simulink model "Model_14Bus_AC_DC_Microgrid"  (R2025a)
settings: Solver=ode23tb  StartTime=0.0  StopTime=0.1  MaxStep=1e-2  RelTol=1e-3
InitFcn:
  | Set_parameters_R2018
StopFcn:
  | Save_Data;
  | Graphics;
undefined symbols (not defined in the file): Clink, D1, Delta, dis1, dis10, dis11, dis12, dis13, dis14, dis2, dis3, dis4, dis5, dis6, dis7, dis8, dis9, Fc, Fnom, Hydride, Increment_MPPT, Ion, Ki_Ireg, Ki_VDCreg, Kp_Ireg, Kp_VDCreg, LimitL_Ireg, LimitL_VDCreg, Limits_MPPT, LimitU_Ireg, LimitU_VDCreg, Lithium, max_min, Metal, Nickel, P_Load_2, P_Load_3, Pnom, Pnom_T1, Pnom_T2, Pnom_T3, Pnom_xfo, Ql_Load_2, Ql_Load_3, R_Load_9, R_Load_DC, RL, Rl, RLff, Rls, sigbuilder_block, Ts, Ts_Control, Ts_Power, V1_LL_T3, Vf, Vfd, Vnom_dc, Vnom_DC, Vnom_Diesel ... (+5)
libraries: spsRMSLib x87, spsCurrentMeasurementLib x47, spsThreePhaseVIMeasurementLib x23, spsVoltageMeasurementLib x21, spsPowerLib x21, spsTHDLib x20, spsThreePhaseSeriesRLCBranchLib x20, spsSeriesRLCBranchLib x19, spsIGBTDiodeLib x14, spsThreePhaseBreakerLib x14, powerlib_extras x14, simulink x12
(part 3 of 9)

== system Model_14Bus_AC_DC_Microgrid/Bus_14 9 ==
  " r1_ L13" : Constant  Value=Rl
  Active powers losses A : Display
      settings: Format=bank
  Active powers losses B : Display
      settings: Format=bank
  Active powers losses c : Display
      settings: Format=bank
  "Delta Pabc " : Scope  NumInputPorts=4
      settings: SampleTime=Ts  Title=Active powers losses A (kW)  ActiveDisplayYMinimum=-0.00443  ActiveDisplayYMaximum=0.03985  DataLoggingSaveFormat=Array
  Math Function : Math  Operator=square  SignedPower=on
  Math Function1 : Math  Operator=square  SignedPower=on
  Math Function2 : Math  Operator=square  SignedPower=on
  Mux : Mux  Inputs=3
  Product : Product
  Product1 : Product
  Product2 : Product
  RMS1 : spsRMSLib/RMS  TrueRMS=on  Freq=60  RMSInit=0  Ts=0
  RMS2 : spsRMSLib/RMS  TrueRMS=on  Freq=60  RMSInit=0  Ts=0
  RMS3 : spsRMSLib/RMS  TrueRMS=on  Freq=60  RMSInit=0  Ts=0
  W_to_kW : Gain  Gain=1e-3
  W_to_kW1 : Gain  Gain=1e-3
  W_to_kW2 : Gain  Gain=1e-3
  tag scope: Power_Losse_abc_L8=global
  wires:
  Math Function/1 -> Product/2
  [Ia_L8] -> RMS2/1
  Math Function1/1 -> Product1/2
  [Ib_L8] -> RMS1/1
  Math Function2/1 -> Product2/2
  " r1_ L13"/1 -> Product2/1, Product1/1, Product/1
  [Ic_L8] -> RMS3/1
  Product/1 -> W_to_kW/1
  Product2/1 -> W_to_kW2/1
  Product1/1 -> W_to_kW1/1
  RMS2/1 -> Math Function/1
  RMS1/1 -> Math Function1/1
  RMS3/1 -> Math Function2/1
  W_to_kW/1 -> Mux/1, "Delta Pabc "/1, Active powers losses A/1  "D_Pa_kW"
  W_to_kW1/1 -> Mux/2, "Delta Pabc "/2, Active powers losses B/1  "D_Pb_kW"
  W_to_kW2/1 -> Active powers losses c/1, Mux/3, "Delta Pabc "/3  "D_Pc_kW"
  Mux/1 -> [Power_Losse_abc_L8], "Delta Pabc "/4

== system Model_14Bus_AC_DC_Microgrid/Bus_2 ==
  note: C
  note: B
  note: A
  note: A
  note: B
  note: Linea - Neutro
  note: C
  note: A
  note: B
  note: C
  Conv pu1 : Gain  Gain=sqrt (3) /Vnom_sec  SaturateOnIntegerOverflow=on  OutDataTypeStr=Inherit: Same as input  ParamDataTypeStr=Inherit: Same as input
  Conv pu2 : Gain  Gain=sqrt (3) /Vnom_sec  SaturateOnIntegerOverflow=on  OutDataTypeStr=Inherit: Same as input  ParamDataTypeStr=Inherit: Same as input
  Measurement1 : Scope  NumInputPorts=4
      settings: SampleTime=Ts  Title=Active Powers (W)  ActiveDisplayYMinimum=-7513.46294  ActiveDisplayYMaximum=8729.48723  DataLoggingVariableName=ScopeData7  DataLoggingSaveFormat=Array
  PLL : Subsystem
  PLL (3ph) : spsPLL3phLib/PLL (3ph)  Fmin=45  Par_Init=[0, 60]  ParK=[180, 3200, 1]  TcD=1e-4  MaxRateChangeFreq=12  FilterCutOffFreq=25  Ts=0  AGC=on
  Power Factor Block1 : Subsystem  mask(Power Factor Block){Freq=Fnom, Vinit=[0, 0], Iinit=[0, 0], Ts=0}
      mask prompts: Freq "Fundamental frequency (Hz):"; Vinit "Voltage initial input [ Mag, Phase (degrees) ]:"; Iinit "Current initial input [ Mag, Phase (degrees) ]:"; Ts "Sample time:"
      mask help:
      | Power Factor Block developed by Dr Rodney Tan
      | Version 1.01 (Aug 2016)
      |
      | Compute power factor and phase angle of AC circuit voltage-current pair at fundamental frequency.
      |
      | The computation is based on Power block and Complex number function block.
      |
      | For the first cycle of simulation, the outputs are held constant to the powers computed for the Voltage initial input and Current initial input parameters.
      mask Help:
      | <b>Fundamental Frequency (Hz)</b>
      | Specify the measurement fundamental frequency, in hertz, of the input signal.
      | 
      | <b>Voltage initial input [ Mag, Phase (degrees) ]</b>
      | Specify the voltage initial magnitude and phase to set a constant output for the first cycle of simulation.
      | 
      | <b>Current initial input [ Mag, Phase (degrees) ]</b>
      | Specify the current initial magnitude and phase to set a constant output for the first cycle of simulation.
      | 
      | <b>Sample Time</b>
      | Specify the sample time of the block, in seconds. Set to 0 to implement a continuous block.
      mask TypeOptions Freq: Power/Freq
      mask TypeOptions Vinit: Power/Vinit
      mask TypeOptions Iinit: Power/Iinit
      mask TypeOptions Ts: Power/Ts
  Power Factor1 : Display
  Scope : Scope
      settings: ActiveDisplayYMinimum=-60.00715  ActiveDisplayYMaximum=239.87716
  Scope2 : Scope
      settings: DataLoggingVariableName=ScopeData8
  THD : spsTHDLib/THD  Freq=60  Ts=Ts_Power
  THD (% and signal) : Scope  NumInputPorts=2
      settings: TimeSpan=0.1  ActiveDisplayYMinimum=-187.16352  ActiveDisplayYMaximum=186.2085  DataLoggingVariableName=ScopeData14
  THD (%) : Display
      settings: Format=bank
  Terminator : Terminator
  Vabc pu1 : Scope
      settings: TimeSpan=3  Title=Vabc_Instantaneo y rms (pu)  ActiveDisplayYMinimum=-2.1863  ActiveDisplayYMaximum=2.45758  DataLoggingVariableName=ScopeData9
  frecuency (Hz) : Display
  to % : Gain  Gain=100  SampleTime=Ts_Power
  ángulo de V (%)1 : Display
      settings: Format=bank
  tag scope: PFabc_Bus2=global, THDv_abc_Bus2=global, delta_abc_Bus2=global
  wires:
  [IabcLL_Bus_2] -> Power Factor Block1/2(Iabc)
  THD/1 -> to %/1
  Power Factor Block1/3(Vabc y Vabc (rms)) -> Conv pu1/1, Measurement1/3
  Power Factor Block1/4(Iabc y Iabc (rms)) -> Measurement1/4
  Conv pu1/1 -> Vabc pu1/1
  Power Factor Block1/2(Qabc) -> Measurement1/2
  Power Factor Block1/1(Pabc) -> Measurement1/1
  Power Factor Block1/5("PFabc ") -> [PFabc_Bus2], Power Factor1/1
  to %/1 -> [THDv_abc_Bus2], THD (%)/1, THD (% and signal)/2  "THD (%)"
  Conv pu2/1 -> PLL/1(Vabc_LN_pu)
  PLL/1(delta_abc) -> [delta_abc_Bus2], Scope/1, ángulo de V (%)1/1
  PLL (3ph)/2 -> Terminator/1
  [VabcLL_Bus_2] -> PLL (3ph)/1, Conv pu2/1, THD/1, THD (% and signal)/1, Power Factor Block1/1(Vabc)  "Vabc"
  PLL (3ph)/1 -> Scope2/1, frecuency (Hz)/1

== system Model_14Bus_AC_DC_Microgrid/Bus_3 ==
  note: C
  note: B
  note: A
  note: C
  note: Linea - Neutro
  note: B
  note: A
  note: A
  note: B
  note: C
  Conv pu1 : Gain  Gain=sqrt (3) /Vnom_sec  SaturateOnIntegerOverflow=on  OutDataTypeStr=Inherit: Same as input  ParamDataTypeStr=Inherit: Same as input
  Conv pu2 : Gain  Gain=sqrt (3) /Vnom_sec  SaturateOnIntegerOverflow=on  OutDataTypeStr=Inherit: Same as input  ParamDataTypeStr=Inherit: Same as input
  Measurement1 : Scope  NumInputPorts=4
      settings: SampleTime=Ts  Title=Active Powers (W)  ActiveDisplayYMinimum=-2991.72001  ActiveDisplayYMaximum=26925.48012  DataLoggingVariableName=ScopeData15  DataLoggingSaveFormat=Array
  PLL : Subsystem
  Power Factor Block1 : Subsystem  mask(Power Factor Block){Freq=Fnom, Vinit=[0, 0], Iinit=[0, 0], Ts=0}
      mask prompts: Freq "Fundamental frequency (Hz):"; Vinit "Voltage initial input [ Mag, Phase (degrees) ]:"; Iinit "Current initial input [ Mag, Phase (degrees) ]:"; Ts "Sample time:"
      mask help:
      | Power Factor Block developed by Dr Rodney Tan
      | Version 1.01 (Aug 2016)
      |
      | Compute power factor and phase angle of AC circuit voltage-current pair at fundamental frequency.
      |
      | The computation is based on Power block and Complex number function block.
      |
      | For the first cycle of simulation, the outputs are held constant to the powers computed for the Voltage initial input and Current initial input parameters.
      mask Help:
      | <b>Fundamental Frequency (Hz)</b>
      | Specify the measurement fundamental frequency, in hertz, of the input signal.
      | 
      | <b>Voltage initial input [ Mag, Phase (degrees) ]</b>
      | Specify the voltage initial magnitude and phase to set a constant output for the first cycle of simulation.
      | 
      | <b>Current initial input [ Mag, Phase (degrees) ]</b>
      | Specify the current initial magnitude and phase to set a constant output for the first cycle of simulation.
      | 
      | <b>Sample Time</b>
      | Specify the sample time of the block, in seconds. Set to 0 to implement a continuous block.
      mask TypeOptions Freq: Power/Freq
      mask TypeOptions Vinit: Power/Vinit
      mask TypeOptions Iinit: Power/Iinit
      mask TypeOptions Ts: Power/Ts
  Power Factor1 : Display
  Scope : Scope
      settings: ActiveDisplayYMinimum=-60.00715  ActiveDisplayYMaximum=239.87716  DataLoggingVariableName=ScopeData2
  THD : spsTHDLib/THD  Freq=60  Ts=Ts_Power
  THD (% and signal) : Scope  NumInputPorts=2
      settings: TimeSpan=0.1  ActiveDisplayYMinimum=-21318.64578  ActiveDisplayYMaximum=21318.87173  DataLoggingVariableName=ScopeData15
  THD (%) : Display
      settings: Format=bank
  Vabc pu1 : Scope
      settings: TimeSpan=3  Title=Vabc_Instantaneo y rms (pu)  ActiveDisplayYMinimum=-2.20522  ActiveDisplayYMaximum=2.66794  DataLoggingVariableName=ScopeData16
  to % : Gain  Gain=100  SampleTime=Ts_Power
  ángulo de V (%)1 : Display
      settings: Format=bank
  tag scope: PFabc_Bus3=global, THDv_abc_Bus3=global, delta_abc_Bus3=global
  wires:
  [IabcLL_Bus_3] -> Power Factor Block1/2(Iabc)
  THD/1 -> to %/1
  Power Factor Block1/4(Iabc y Iabc (rms)) -> Measurement1/4
  Power Factor Block1/1(Pabc) -> Measurement1/1
  Conv pu1/1 -> Vabc pu1/1
  Power Factor Block1/2(Qabc) -> Measurement1/2
  Power Factor Block1/3(Vabc y Vabc (rms)) -> Conv pu1/1, Measurement1/3
  Power Factor Block1/5("PFabc ") -> [PFabc_Bus3], Power Factor1/1
  to %/1 -> [THDv_abc_Bus3], THD (%)/1, THD (% and signal)/2  "THD (%)"
  Conv pu2/1 -> PLL/1(Vabc_LN_pu)
  PLL/1(delta_abc) -> [delta_abc_Bus3], Scope/1, ángulo de V (%)1/1
  [VabcLL_Bus_3] -> Conv pu2/1, THD/1, THD (% and signal)/1, Power Factor Block1/1(Vabc)  "Signal Vabc"

== system Model_14Bus_AC_DC_Microgrid/Bus_4 ==
  note: C
  note: B
  note: A
  note: C
  note: Linea - Neutro
  note: B
  note: A
  note: A
  note: B
  note: C
  Conv pu1 : Gain  Gain=sqrt (3) /Vnom_sec  SaturateOnIntegerOverflow=on  OutDataTypeStr=Inherit: Same as input  ParamDataTypeStr=Inherit: Same as input
  Conv pu2 : Gain  Gain=sqrt (3) /Vnom_sec  SaturateOnIntegerOverflow=on  OutDataTypeStr=Inherit: Same as input  ParamDataTypeStr=Inherit: Same as input
  Measurement1 : Scope  NumInputPorts=4
      settings: SampleTime=Ts  Title=Active Powers (W)  ActiveDisplayYMinimum=-5628.05752  ActiveDisplayYMaximum=50652.51771  DataLoggingVariableName=ScopeData23  DataLoggingSaveFormat=Array
  PLL : Subsystem
  Power Factor Block1 : Subsystem  mask(Power Factor Block){Freq=Fnom, Vinit=[0, 0], Iinit=[0, 0], Ts=0}
      mask prompts: Freq "Fundamental frequency (Hz):"; Vinit "Voltage initial input [ Mag, Phase (degrees) ]:"; Iinit "Current initial input [ Mag, Phase (degrees) ]:"; Ts "Sample time:"
      mask help:
      | Power Factor Block developed by Dr Rodney Tan
      | Version 1.01 (Aug 2016)
      |
      | Compute power factor and phase angle of AC circuit voltage-current pair at fundamental frequency.
      |
      | The computation is based on Power block and Complex number function block.
      |
      | For the first cycle of simulation, the outputs are held constant to the powers computed for the Voltage initial input and Current initial input parameters.
      mask Help:
      | <b>Fundamental Frequency (Hz)</b>
      | Specify the measurement fundamental frequency, in hertz, of the input signal.
      | 
      | <b>Voltage initial input [ Mag, Phase (degrees) ]</b>
      | Specify the voltage initial magnitude and phase to set a constant output for the first cycle of simulation.
      | 
      | <b>Current initial input [ Mag, Phase (degrees) ]</b>
      | Specify the current initial magnitude and phase to set a constant output for the first cycle of simulation.
      | 
      | <b>Sample Time</b>
      | Specify the sample time of the block, in seconds. Set to 0 to implement a continuous block.
      mask TypeOptions Freq: Power/Freq
      mask TypeOptions Vinit: Power/Vinit
      mask TypeOptions Iinit: Power/Iinit
      mask TypeOptions Ts: Power/Ts
  Power Factor1 : Display
  Scope : Scope
      settings: ActiveDisplayYMinimum=-60.00715  ActiveDisplayYMaximum=239.87716  DataLoggingVariableName=ScopeData3
  THD : spsTHDLib/THD  Freq=60  Ts=Ts_Power
  THD (% and signal) : Scope  NumInputPorts=2
      settings: TimeSpan=0.1  ActiveDisplayYMinimum=-21318.64578  ActiveDisplayYMaximum=21318.87173  DataLoggingVariableName=ScopeData11
  THD (%) : Display
      settings: Format=bank
  Vabc pu1 : Scope
      settings: TimeSpan=3  Title=Vabc_Instantaneo y rms (pu)  ActiveDisplayYMinimum=-1.73092  ActiveDisplayYMaximum=1.73065  DataLoggingVariableName=ScopeData24
  to % : Gain  Gain=100  SampleTime=Ts_Power
  ángulo de V (%)1 : Display
      settings: Format=bank
  tag scope: PFabc_Bus4=global, THDv_abc_Bus4=global, delta_abc_Bus4=global
  wires:
  [IabcLL_Bus_4] -> Power Factor Block1/2(Iabc)
  THD/1 -> to %/1
  Power Factor Block1/4(Iabc y Iabc (rms)) -> Measurement1/4
  Power Factor Block1/1(Pabc) -> Measurement1/1
  Conv pu1/1 -> Vabc pu1/1
  Power Factor Block1/2(Qabc) -> Measurement1/2
  Power Factor Block1/3(Vabc y Vabc (rms)) -> Conv pu1/1, Measurement1/3
  Power Factor Block1/5("PFabc ") -> [PFabc_Bus4], Power Factor1/1
  to %/1 -> [THDv_abc_Bus4], THD (%)/1, THD (% and signal)/2  "THD (%)"
  Conv pu2/1 -> PLL/1(Vabc_LN_pu)
  PLL/1(delta_abc) -> [delta_abc_Bus4], Scope/1, ángulo de V (%)1/1
  [VabcLL_Bus_4] -> Power Factor Block1/1(Vabc), Conv pu2/1, THD/1, THD (% and signal)/1  "Signal Vabc"

== system Model_14Bus_AC_DC_Microgrid/Bus_5 ==
  note: C
  note: B
  note: A
  note: C
  note: Linea - Neutro
  note: B
  note: A
  note: A
  note: B
  note: C
  Conv pu1 : Gain  Gain=sqrt (3) /Vnom_sec  SaturateOnIntegerOverflow=on  OutDataTypeStr=Inherit: Same as input  ParamDataTypeStr=Inherit: Same as input
  Conv pu2 : Gain  Gain=sqrt (3) /Vnom_sec  SaturateOnIntegerOverflow=on  OutDataTypeStr=Inherit: Same as input  ParamDataTypeStr=Inherit: Same as input
  Measurement1 : Scope  NumInputPorts=4
      settings: SampleTime=Ts  Title=Active Powers (W)  ActiveDisplayYMinimum=-5617.14466  ActiveDisplayYMaximum=50554.30195  DataLoggingVariableName=ScopeData19  DataLoggingSaveFormat=Array
  PLL : Subsystem
  Power Factor Block1 : Subsystem  mask(Power Factor Block){Freq=Fnom, Vinit=[0, 0], Iinit=[0, 0], Ts=0}
      mask prompts: Freq "Fundamental frequency (Hz):"; Vinit "Voltage initial input [ Mag, Phase (degrees) ]:"; Iinit "Current initial input [ Mag, Phase (degrees) ]:"; Ts "Sample time:"
      mask help:
      | Power Factor Block developed by Dr Rodney Tan
      | Version 1.01 (Aug 2016)
      |
      | Compute power factor and phase angle of AC circuit voltage-current pair at fundamental frequency.
      |
      | The computation is based on Power block and Complex number function block.
      |
      | For the first cycle of simulation, the outputs are held constant to the powers computed for the Voltage initial input and Current initial input parameters.
      mask Help:
      | <b>Fundamental Frequency (Hz)</b>
      | Specify the measurement fundamental frequency, in hertz, of the input signal.
      | 
      | <b>Voltage initial input [ Mag, Phase (degrees) ]</b>
      | Specify the voltage initial magnitude and phase to set a constant output for the first cycle of simulation.
      | 
      | <b>Current initial input [ Mag, Phase (degrees) ]</b>
      | Specify the current initial magnitude and phase to set a constant output for the first cycle of simulation.
      | 
      | <b>Sample Time</b>
      | Specify the sample time of the block, in seconds. Set to 0 to implement a continuous block.
      mask TypeOptions Freq: Power/Freq
      mask TypeOptions Vinit: Power/Vinit
      mask TypeOptions Iinit: Power/Iinit
      mask TypeOptions Ts: Power/Ts
  Power Factor1 : Display
  Scope : Scope
      settings: ActiveDisplayYMinimum=-60.00715  ActiveDisplayYMaximum=239.87716  DataLoggingVariableName=ScopeData4
  THD : spsTHDLib/THD  Freq=60  Ts=Ts_Power
  THD (% and signal) : Scope  NumInputPorts=2
      settings: TimeSpan=0.1  ActiveDisplayYMinimum=-363.53745  ActiveDisplayYMaximum=363.57971  DataLoggingVariableName=ScopeData12
  THD (%) : Display
      settings: Format=bank
  Vabc pu1 : Scope
      settings: TimeSpan=3  Title=Vabc_Instantaneo y rms (pu)  ActiveDisplayYMinimum=-1.78329  ActiveDisplayYMaximum=1.78457  DataLoggingVariableName=ScopeData20
  to % : Gain  Gain=100  SampleTime=Ts_Power
  ángulo de V (%)1 : Display
      settings: Format=bank
  tag scope: PFabc_Bus5=global, THDv_abc_Bus5=global, delta_abc_Bus5=global
  wires:
  [IabcLL_Bus_5] -> Power Factor Block1/2(Iabc)
  THD/1 -> to %/1
  Power Factor Block1/4(Iabc y Iabc (rms)) -> Measurement1/4
  Power Factor Block1/1(Pabc) -> Measurement1/1
  Conv pu1/1 -> Vabc pu1/1
  Power Factor Block1/2(Qabc) -> Measurement1/2
  Power Factor Block1/3(Vabc y Vabc (rms)) -> Conv pu1/1, Measurement1/3
  Power Factor Block1/5("PFabc ") -> [PFabc_Bus5], Power Factor1/1
  to %/1 -> [THDv_abc_Bus5], THD (%)/1, THD (% and signal)/2  "THD (%)"
  Conv pu2/1 -> PLL/1(Vabc_LN_pu)
  PLL/1(delta_abc) -> [delta_abc_Bus5], Scope/1, ángulo de V (%)1/1
  [VabcLL_Bus_5] -> Power Factor Block1/1(Vabc), Conv pu2/1, THD/1, THD (% and signal)/1  "Signal Vabc"

== system Model_14Bus_AC_DC_Microgrid/Bus_6  ==
  note: C
  note: B
  note: A
  note: C
  note: Linea - Neutro
  note: B
  note: A
  note: A
  note: B
  Conv pu1 : Gain  Gain=sqrt (3) /Vnom_prim  SaturateOnIntegerOverflow=on  OutDataTypeStr=Inherit: Same as input  ParamDataTypeStr=Inherit: Same as input
  Conv pu2 : Gain  Gain=sqrt (3) /Vnom_prim  SaturateOnIntegerOverflow=on  OutDataTypeStr=Inherit: Same as input  ParamDataTypeStr=Inherit: Same as input
  Measurement1 : Scope  NumInputPorts=4
      settings: SampleTime=Ts  Title=Active Powers (W)  ActiveDisplayYMinimum=-36639.89993  ActiveDisplayYMaximum=329759.09935  DataLoggingVariableName=ScopeData27  DataLoggingSaveFormat=Array
  PLL : Subsystem
  PLL (3ph) : spsPLL3phLib/PLL (3ph)  Fmin=45  Par_Init=[0, 60]  ParK=[180, 3200, 1]  TcD=1e-4  MaxRateChangeFreq=12  FilterCutOffFreq=25  Ts=0  AGC=on
  Power Factor Block1 : Subsystem  mask(Power Factor Block){Freq=Fnom, Vinit=[0, 0], Iinit=[0, 0], Ts=0}
      mask prompts: Freq "Fundamental frequency (Hz):"; Vinit "Voltage initial input [ Mag, Phase (degrees) ]:"; Iinit "Current initial input [ Mag, Phase (degrees) ]:"; Ts "Sample time:"
      mask help:
      | Power Factor Block developed by Dr Rodney Tan
      | Version 1.01 (Aug 2016)
      |
      | Compute power factor and phase angle of AC circuit voltage-current pair at fundamental frequency.
      |
      | The computation is based on Power block and Complex number function block.
      |
      | For the first cycle of simulation, the outputs are held constant to the powers computed for the Voltage initial input and Current initial input parameters.
      mask Help:
      | <b>Fundamental Frequency (Hz)</b>
      | Specify the measurement fundamental frequency, in hertz, of the input signal.
      | 
      | <b>Voltage initial input [ Mag, Phase (degrees) ]</b>
      | Specify the voltage initial magnitude and phase to set a constant output for the first cycle of simulation.
      | 
      | <b>Current initial input [ Mag, Phase (degrees) ]</b>
      | Specify the current initial magnitude and phase to set a constant output for the first cycle of simulation.
      | 
      | <b>Sample Time</b>
      | Specify the sample time of the block, in seconds. Set to 0 to implement a continuous block.
      mask TypeOptions Freq: Power/Freq
      mask TypeOptions Vinit: Power/Vinit
      mask TypeOptions Iinit: Power/Iinit
      mask TypeOptions Ts: Power/Ts
  Power Factor1 : Display
  Scope : Scope
      settings: ActiveDisplayYMinimum=-60.00715  ActiveDisplayYMaximum=239.87716  DataLoggingVariableName=ScopeData8
  Scope2 : Scope
      settings: DataLoggingVariableName=ScopeData6
  THD : spsTHDLib/THD  Freq=60  Ts=Ts_Power
  THD (% and signal) : Scope  NumInputPorts=2
      settings: TimeSpan=0.1  ActiveDisplayYMinimum=-21318.64578  ActiveDisplayYMaximum=21318.87173  DataLoggingVariableName=ScopeData10
  THD (%) : Display
      settings: Format=bank
  Terminator : Terminator
  Vabc pu1 : Scope
      settings: TimeSpan=3  Title=Vabc_Instantaneo y rms (pu)  ActiveDisplayYMinimum=-1.94697  ActiveDisplayYMaximum=2.40512  DataLoggingVariableName=ScopeData28
  frecuency (Hz) : Display
  to % : Gain  Gain=100  SampleTime=Ts_Power
  ángulo de V (%)1 : Display
      settings: Format=bank
  tag scope: PFabc_Bus6=global, THDv_abc_Bus6=global, delta_abc_Bus6=global
  wires:
  [IabcLL_Bus_6] -> Power Factor Block1/2(Iabc)
  THD/1 -> to %/1
  Power Factor Block1/4(Iabc y Iabc (rms)) -> Measurement1/4
  Power Factor Block1/1(Pabc) -> Measurement1/1
  Conv pu1/1 -> Vabc pu1/1
  Power Factor Block1/2(Qabc) -> Measurement1/2
  Power Factor Block1/3(Vabc y Vabc (rms)) -> Conv pu1/1, Measurement1/3
  Power Factor Block1/5("PFabc ") -> [PFabc_Bus6], Power Factor1/1
  to %/1 -> [THDv_abc_Bus6], THD (%)/1, THD (% and signal)/2  "THD (%)"
  PLL/1(delta_abc) -> [delta_abc_Bus6], Scope/1, ángulo de V (%)1/1
  Conv pu2/1 -> PLL/1(Vabc_LN_pu)
  PLL (3ph)/2 -> Terminator/1
  [VabcLL_Bus_6] -> Power Factor Block1/1(Vabc), Conv pu2/1, PLL (3ph)/1, THD/1, THD (% and signal)/1  "Vabc"
  PLL (3ph)/1 -> Scope2/1, frecuency (Hz)/1

== system Model_14Bus_AC_DC_Microgrid/Bus_7 ==
  note: C
  note: B
  note: A
  note: C
  note: Linea - Neutro
  note: B
  note: A
  note: A
  note: B
  Conv pu1 : Gain  Gain=sqrt (3) /Vnom_prim  SaturateOnIntegerOverflow=on  OutDataTypeStr=Inherit: Same as input  ParamDataTypeStr=Inherit: Same as input
  Conv pu2 : Gain  Gain=sqrt (3) /Vnom_prim  SaturateOnIntegerOverflow=on  OutDataTypeStr=Inherit: Same as input  ParamDataTypeStr=Inherit: Same as input
  Measurement1 : Scope  NumInputPorts=4
      settings: SampleTime=Ts  Title=Active Powers (W)  ActiveDisplayYMinimum=-12763.51885  ActiveDisplayYMaximum=112438.93052  DataLoggingVariableName=ScopeData29  DataLoggingSaveFormat=Array
  PLL : Subsystem
  PLL (3ph) : spsPLL3phLib/PLL (3ph)  Fmin=45  Par_Init=[0, 60]  ParK=[180, 3200, 1]  TcD=1e-4  MaxRateChangeFreq=12  FilterCutOffFreq=25  Ts=0  AGC=on
  Power Factor Block1 : Subsystem  mask(Power Factor Block){Freq=Fnom, Vinit=[0, 0], Iinit=[0, 0], Ts=0}
      mask prompts: Freq "Fundamental frequency (Hz):"; Vinit "Voltage initial input [ Mag, Phase (degrees) ]:"; Iinit "Current initial input [ Mag, Phase (degrees) ]:"; Ts "Sample time:"
      mask help:
      | Power Factor Block developed by Dr Rodney Tan
      | Version 1.01 (Aug 2016)
      |
      | Compute power factor and phase angle of AC circuit voltage-current pair at fundamental frequency.
      |
      | The computation is based on Power block and Complex number function block.
      |
      | For the first cycle of simulation, the outputs are held constant to the powers computed for the Voltage initial input and Current initial input parameters.
      mask Help:
      | <b>Fundamental Frequency (Hz)</b>
      | Specify the measurement fundamental frequency, in hertz, of the input signal.
      | 
      | <b>Voltage initial input [ Mag, Phase (degrees) ]</b>
      | Specify the voltage initial magnitude and phase to set a constant output for the first cycle of simulation.
      | 
      | <b>Current initial input [ Mag, Phase (degrees) ]</b>
      | Specify the current initial magnitude and phase to set a constant output for the first cycle of simulation.
      | 
      | <b>Sample Time</b>
      | Specify the sample time of the block, in seconds. Set to 0 to implement a continuous block.
      mask TypeOptions Freq: Power/Freq
      mask TypeOptions Vinit: Power/Vinit
      mask TypeOptions Iinit: Power/Iinit
      mask TypeOptions Ts: Power/Ts
  Power Factor1 : Display
  Scope : Scope
      settings: ActiveDisplayYMinimum=-55.0107  ActiveDisplayYMaximum=235.47977  DataLoggingVariableName=ScopeData9
  Scope2 : Scope
      settings: DataLoggingVariableName=ScopeData2
  THD : spsTHDLib/THD  Freq=60  Ts=Ts_Power
  THD (% and signal) : Scope  NumInputPorts=2
      settings: TimeSpan=0.1  ActiveDisplayYMinimum=-21318.64578  ActiveDisplayYMaximum=21318.87173  DataLoggingVariableName=ScopeData6
  THD (%) : Display
      settings: Format=bank
  Terminator : Terminator
  Vabc pu1 : Scope
      settings: TimeSpan=3  Title=Vabc_Instantaneo y rms (pu)  ActiveDisplayYMinimum=-1.7414  ActiveDisplayYMaximum=1.74142  DataLoggingVariableName=ScopeData30
  frecuency (Hz) : Display
  to % : Gain  Gain=100  SampleTime=Ts_Power
  ángulo de V (%)1 : Display
      settings: Format=bank
  tag scope: PFabc_Bus7=global, THDv_abc_Bus7=global, delta_abc_Bus7=global
  wires:
  [IabcLL_Bus_7] -> Power Factor Block1/2(Iabc)
  THD/1 -> to %/1
  Power Factor Block1/4(Iabc y Iabc (rms)) -> Measurement1/4
  Power Factor Block1/1(Pabc) -> Measurement1/1
  Conv pu1/1 -> Vabc pu1/1
  Power Factor Block1/2(Qabc) -> Measurement1/2
  Power Factor Block1/3(Vabc y Vabc (rms)) -> Conv pu1/1, Measurement1/3
  to %/1 -> [THDv_abc_Bus7], THD (%)/1, THD (% and signal)/2  "THD (%)"
  Power Factor Block1/5("PFabc ") -> [PFabc_Bus7], Power Factor1/1
  PLL/1(delta_abc) -> [delta_abc_Bus7], Scope/1, ángulo de V (%)1/1
  Conv pu2/1 -> PLL/1(Vabc_LN_pu)
  [VabcLL_Bus_7] -> PLL (3ph)/1, Conv pu2/1, THD/1, THD (% and signal)/1, Power Factor Block1/1(Vabc)  "Vabc"
  PLL (3ph)/2 -> Terminator/1
  PLL (3ph)/1 -> Scope2/1, frecuency (Hz)/1

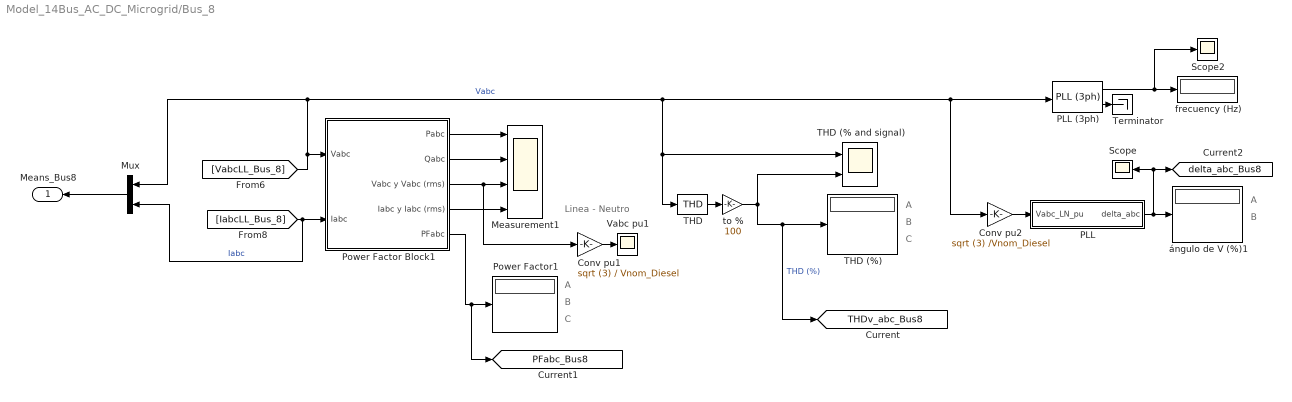
== system Model_14Bus_AC_DC_Microgrid/Bus_8       ==
  note: C
  note: B
  note: A
  note: C
  note: Linea - Neutro
  note: B
  note: A
  note: A
  note: B
  Conv pu1 : Gain  Gain=sqrt (3) / Vnom_Diesel  SaturateOnIntegerOverflow=on  OutDataTypeStr=Inherit: Same as input  ParamDataTypeStr=Inherit: Same as input
  Conv pu2 : Gain  Gain=sqrt (3) /Vnom_Diesel  SaturateOnIntegerOverflow=on  OutDataTypeStr=Inherit: Same as input  ParamDataTypeStr=Inherit: Same as input
  Measurement1 : Scope  NumInputPorts=4
      settings: SampleTime=Ts  Title=Active Powers (W)  ActiveDisplayYMinimum=-14254.34196  ActiveDisplayYMaximum=128289.07765  DataLoggingVariableName=ScopeData25  DataLoggingSaveFormat=Array
  Mux : Mux  Inputs=2
  PLL : Subsystem
  PLL (3ph) : spsPLL3phLib/PLL (3ph)  Fmin=45  Par_Init=[0, 60]  ParK=[180, 3200, 1]  TcD=1e-4  MaxRateChangeFreq=12  FilterCutOffFreq=25  Ts=0  AGC=on
  Power Factor Block1 : Subsystem  mask(Power Factor Block){Freq=Fnom, Vinit=[0, 0], Iinit=[0, 0], Ts=0}
      mask prompts: Freq "Fundamental frequency (Hz):"; Vinit "Voltage initial input [ Mag, Phase (degrees) ]:"; Iinit "Current initial input [ Mag, Phase (degrees) ]:"; Ts "Sample time:"
      mask help:
      | Power Factor Block developed by Dr Rodney Tan
      | Version 1.01 (Aug 2016)
      |
      | Compute power factor and phase angle of AC circuit voltage-current pair at fundamental frequency.
      |
      | The computation is based on Power block and Complex number function block.
      |
      | For the first cycle of simulation, the outputs are held constant to the powers computed for the Voltage initial input and Current initial input parameters.
      mask Help:
      | <b>Fundamental Frequency (Hz)</b>
      | Specify the measurement fundamental frequency, in hertz, of the input signal.
      | 
      | <b>Voltage initial input [ Mag, Phase (degrees) ]</b>
      | Specify the voltage initial magnitude and phase to set a constant output for the first cycle of simulation.
      | 
      | <b>Current initial input [ Mag, Phase (degrees) ]</b>
      | Specify the current initial magnitude and phase to set a constant output for the first cycle of simulation.
      | 
      | <b>Sample Time</b>
      | Specify the sample time of the block, in seconds. Set to 0 to implement a continuous block.
      mask TypeOptions Freq: Power/Freq
      mask TypeOptions Vinit: Power/Vinit
      mask TypeOptions Iinit: Power/Iinit
      mask TypeOptions Ts: Power/Ts
  Power Factor1 : Display
  Scope : Scope
      settings: ActiveDisplayYMinimum=-71.81024  ActiveDisplayYMaximum=228.41349  DataLoggingVariableName=ScopeData10
  Scope2 : Scope
  THD : spsTHDLib/THD  Freq=60  Ts=Ts_Power
  THD (% and signal) : Scope  NumInputPorts=2
      settings: TimeSpan=0.1  ActiveDisplayYMinimum=-21318.64578  ActiveDisplayYMaximum=21318.87173  DataLoggingVariableName=ScopeData7
  THD (%) : Display
      settings: Format=bank
  Terminator : Terminator
  Vabc pu1 : Scope
      settings: TimeSpan=3  Title=Vabc_Instantaneo y rms (pu)  ActiveDisplayYMinimum=-2.44601  ActiveDisplayYMaximum=2.65682  DataLoggingVariableName=ScopeData26
  frecuency (Hz) : Display
  to % : Gain  Gain=100  SampleTime=Ts_Power
  ángulo de V (%)1 : Display
      settings: Format=bank
  "Means_Bus8      " : Outport  VectorParamsAs1DForOutWhenUnconnected=off
  tag scope: PFabc_Bus8=global, THDv_abc_Bus8=global, delta_abc_Bus8=global
  wires:
  [IabcLL_Bus_8] -> Power Factor Block1/2(Iabc), Mux/2  "Iabc"
  THD/1 -> to %/1
  Mux/1 -> "Means_Bus8      "/1
  Power Factor Block1/4(Iabc y Iabc (rms)) -> Measurement1/4
  Power Factor Block1/1(Pabc) -> Measurement1/1
  Conv pu1/1 -> Vabc pu1/1
  Power Factor Block1/2(Qabc) -> Measurement1/2
  Power Factor Block1/3(Vabc y Vabc (rms)) -> Conv pu1/1, Measurement1/3
  to %/1 -> [THDv_abc_Bus8], THD (%)/1, THD (% and signal)/2  "THD (%)"
  Power Factor Block1/5("PFabc ") -> [PFabc_Bus8], Power Factor1/1
  PLL/1(delta_abc) -> [delta_abc_Bus8], Scope/1, ángulo de V (%)1/1
  Conv pu2/1 -> PLL/1(Vabc_LN_pu)
  PLL (3ph)/2 -> Terminator/1
  PLL (3ph)/1 -> Scope2/1, frecuency (Hz)/1
  [VabcLL_Bus_8] -> Power Factor Block1/1(Vabc), Mux/1, Conv pu2/1, PLL (3ph)/1, THD/1, THD (% and signal)/1  "Vabc"

== system Model_14Bus_AC_DC_Microgrid/Bus_9 ==
  note: C
  note: B
  note: A
  note: C
  note: Linea - Neutro
  note: B
  note: A
  note: A
  note: B
  Conv pu1 : Gain  Gain=sqrt (3) /Vnom_prim  SaturateOnIntegerOverflow=on  OutDataTypeStr=Inherit: Same as input  ParamDataTypeStr=Inherit: Same as input
  Conv pu2 : Gain  Gain=sqrt (3) /Vnom_prim  SaturateOnIntegerOverflow=on  OutDataTypeStr=Inherit: Same as input  ParamDataTypeStr=Inherit: Same as input
  Measurement1 : Scope  NumInputPorts=4
      settings: SampleTime=Ts  Title=Active Powers (W)  ActiveDisplayYMinimum=-33798.98763  ActiveDisplayYMaximum=304190.88869  DataLoggingVariableName=ScopeData37  DataLoggingSaveFormat=Array
  PLL : Subsystem
  Power Factor Block1 : Subsystem  mask(Power Factor Block){Freq=Fnom, Vinit=[0, 0], Iinit=[0, 0], Ts=0}
      mask prompts: Freq "Fundamental frequency (Hz):"; Vinit "Voltage initial input [ Mag, Phase (degrees) ]:"; Iinit "Current initial input [ Mag, Phase (degrees) ]:"; Ts "Sample time:"
      mask help:
      | Power Factor Block developed by Dr Rodney Tan
      | Version 1.01 (Aug 2016)
      |
      | Compute power factor and phase angle of AC circuit voltage-current pair at fundamental frequency.
      |
      | The computation is based on Power block and Complex number function block.
      |
      | For the first cycle of simulation, the outputs are held constant to the powers computed for the Voltage initial input and Current initial input parameters.
      mask Help:
      | <b>Fundamental Frequency (Hz)</b>
      | Specify the measurement fundamental frequency, in hertz, of the input signal.
      | 
      | <b>Voltage initial input [ Mag, Phase (degrees) ]</b>
      | Specify the voltage initial magnitude and phase to set a constant output for the first cycle of simulation.
      | 
      | <b>Current initial input [ Mag, Phase (degrees) ]</b>
      | Specify the current initial magnitude and phase to set a constant output for the first cycle of simulation.
      | 
      | <b>Sample Time</b>
      | Specify the sample time of the block, in seconds. Set to 0 to implement a continuous block.
      mask TypeOptions Freq: Power/Freq
      mask TypeOptions Vinit: Power/Vinit
      mask TypeOptions Iinit: Power/Iinit
      mask TypeOptions Ts: Power/Ts
  Power Factor1 : Display
  Scope : Scope
      settings: ActiveDisplayYMinimum=-60.00715  ActiveDisplayYMaximum=239.87716  DataLoggingVariableName=ScopeData11
  THD : spsTHDLib/THD  Freq=60  Ts=Ts_Power
  THD (% and signal) : Scope  NumInputPorts=2
      settings: TimeSpan=0.1  ActiveDisplayYMinimum=-21318.64578  ActiveDisplayYMaximum=21318.87173  DataLoggingVariableName=ScopeData5
  THD (%) : Display
      settings: Format=bank
  Vabc pu1 : Scope
      settings: TimeSpan=3  Title=Vabc_Instantaneo y rms (pu)  ActiveDisplayYMinimum=-1.92888  ActiveDisplayYMaximum=2.57371  DataLoggingVariableName=ScopeData38
  to % : Gain  Gain=100  SampleTime=Ts_Power
  ángulo de V (%)1 : Display
      settings: Format=bank
  tag scope: PFabc_Bus9=global, THDv_abc_Bus9=global, delta_abc_Bus9=global
  wires:
  [IabcLL_Bus_9] -> Power Factor Block1/2(Iabc)
  THD/1 -> to %/1
  Power Factor Block1/4(Iabc y Iabc (rms)) -> Measurement1/4
  Power Factor Block1/1(Pabc) -> Measurement1/1
  Conv pu1/1 -> Vabc pu1/1
  Power Factor Block1/2(Qabc) -> Measurement1/2
  Power Factor Block1/3(Vabc y Vabc (rms)) -> Conv pu1/1, Measurement1/3
  to %/1 -> [THDv_abc_Bus9], THD (%)/1, THD (% and signal)/2  "THD (%)"
  Power Factor Block1/5("PFabc ") -> [PFabc_Bus9], Power Factor1/1
  PLL/1(delta_abc) -> [delta_abc_Bus9], Scope/1, ángulo de V (%)1/1
  [VabcLL_Bus_9] -> Conv pu2/1, THD/1, THD (% and signal)/1, Power Factor Block1/1(Vabc)  "Signal Vabc"
  Conv pu2/1 -> PLL/1(Vabc_LN_pu)

== system Model_14Bus_AC_DC_Microgrid/Bus_AC PV  ==
  note: C
  note: B
  note: A
  note: C
  note: Linea - Neutro
  note: B
  note: A
  note: B
  note: A
  note: C
  Conv pu1 : Gain  Gain=sqrt (3) /Vnom_prim  SaturateOnIntegerOverflow=on  OutDataTypeStr=Inherit: Same as input  ParamDataTypeStr=Inherit: Same as input
  Conv pu2 : Gain  Gain=sqrt (3) /Vnom_prim  SaturateOnIntegerOverflow=on  OutDataTypeStr=Inherit: Same as input  ParamDataTypeStr=Inherit: Same as input
  Measurement1 : Scope  NumInputPorts=4
      settings: SampleTime=Ts  Title=Active Powers (W)  ActiveDisplayYMinimum=-34723.33435  ActiveDisplayYMaximum=312510.00919  DataLoggingVariableName=ScopeData31  DataLoggingSaveFormat=Array
  PLL : Subsystem
  PLL (3ph) : spsPLL3phLib/PLL (3ph)  Fmin=45  Par_Init=[0, 60]  ParK=[180, 3200, 1]  TcD=1e-4  MaxRateChangeFreq=12  FilterCutOffFreq=25  Ts=0  AGC=on
  Power Factor Block1 : Subsystem  mask(Power Factor Block){Freq=Fnom, Vinit=[0, 0], Iinit=[0, 0], Ts=0}
      mask prompts: Freq "Fundamental frequency (Hz):"; Vinit "Voltage initial input [ Mag, Phase (degrees) ]:"; Iinit "Current initial input [ Mag, Phase (degrees) ]:"; Ts "Sample time:"
      mask help:
      | Power Factor Block developed by Dr Rodney Tan
      | Version 1.01 (Aug 2016)
      |
      | Compute power factor and phase angle of AC circuit voltage-current pair at fundamental frequency.
      |
      | The computation is based on Power block and Complex number function block.
      |
      | For the first cycle of simulation, the outputs are held constant to the powers computed for the Voltage initial input and Current initial input parameters.
      mask Help:
      | <b>Fundamental Frequency (Hz)</b>
      | Specify the measurement fundamental frequency, in hertz, of the input signal.
      | 
      | <b>Voltage initial input [ Mag, Phase (degrees) ]</b>
      | Specify the voltage initial magnitude and phase to set a constant output for the first cycle of simulation.
      | 
      | <b>Current initial input [ Mag, Phase (degrees) ]</b>
      | Specify the current initial magnitude and phase to set a constant output for the first cycle of simulation.
      | 
      | <b>Sample Time</b>
      | Specify the sample time of the block, in seconds. Set to 0 to implement a continuous block.
      mask TypeOptions Freq: Power/Freq
      mask TypeOptions Vinit: Power/Vinit
      mask TypeOptions Iinit: Power/Iinit
      mask TypeOptions Ts: Power/Ts
  Power Factor1 : Display
  Scope : Scope
      settings: ActiveDisplayYMinimum=-56.88569  ActiveDisplayYMaximum=237.8062  DataLoggingVariableName=ScopeData4
  Scope2 : Scope
      settings: DataLoggingVariableName=ScopeData5
  THD : spsTHDLib/THD  Freq=60  Ts=Ts_Power
  THD (% and signal) : Scope  NumInputPorts=2
      settings: TimeSpan=0.1  ActiveDisplayYMinimum=-21318.64578  ActiveDisplayYMaximum=21318.87173  DataLoggingVariableName=ScopeData9
  THD (%) : Display
      settings: Format=bank
  Terminator : Terminator
  Vabc pu1 : Scope
      settings: TimeSpan=3  Title=Vabc_Instantaneo y rms (pu)  ActiveDisplayYMinimum=-1.80551  ActiveDisplayYMaximum=1.80566  DataLoggingVariableName=ScopeData32
  frecuency (Hz) : Display
  to % : Gain  Gain=100  SampleTime=Ts_Power
  ángulo de V (%)1 : Display
      settings: Format=bank
  wires:
  [Iabc_B1] -> Power Factor Block1/2(Iabc)
  THD/1 -> to %/1
  to %/1 -> THD (%)/1, THD (% and signal)/2  "THD (%)"
  Power Factor Block1/4(Iabc y Iabc (rms)) -> Measurement1/4
  Power Factor Block1/1(Pabc) -> Measurement1/1
  Conv pu1/1 -> Vabc pu1/1
  Power Factor Block1/5("PFabc ") -> Power Factor1/1
  Power Factor Block1/2(Qabc) -> Measurement1/2
  Power Factor Block1/3(Vabc y Vabc (rms)) -> Conv pu1/1, Measurement1/3
  Conv pu2/1 -> PLL/1(Vabc_LN_pu)
  PLL/1(delta_abc) -> Scope/1, ángulo de V (%)1/1
  PLL (3ph)/1 -> Scope2/1, frecuency (Hz)/1
  PLL (3ph)/2 -> Terminator/1
  [Vabc_B1] -> Power Factor Block1/1(Vabc), PLL (3ph)/1, Conv pu2/1, THD/1, THD (% and signal)/1  "Vabc"

== system Model_14Bus_AC_DC_Microgrid/Bus_AC//DC3 ==
  note: BUS
  Battery system : Subsystem
      mask Display: disp('Open this block\nto display additional \nscopes & measurements')
  Conv pu1 : Gain  Gain=1 /Vnom_DC  SaturateOnIntegerOverflow=on  OutDataTypeStr=Inherit: Same as input  ParamDataTypeStr=Inherit: Same as input
  Display6 : Display
  Gain : Gain  Gain=-2/1000
  Mean : spsMeanLib/Mean  Freq=10  Vinit=0  Ts=0
  Mux : Mux  Inputs=2
  PV system : Subsystem
      mask Display: disp('Open this block\nto display additional \nscopes & measurements')
  Product : Product
  Scope3 : Scope  NumInputPorts=3
      settings: ActiveDisplayYMinimum=-0.11121  ActiveDisplayYMaximum=1.00094  DataLoggingVariableName=ScopeData20
  tag scope: P_BusDC=global, V_pu_BusDC=global
  wires:
  Conv pu1/1 -> Scope3/1, [V_pu_BusDC]  "DC Voltage (pu)"
  [Vdc_bus] -> Product/1, Conv pu1/1
  [I_BusDC] -> Mux/1, Mean/1  "instant current DC (A)"
  Mean/1 -> Product/2, Mux/2, Display6/1  "Current mean DC (A)"
  Product/1 -> Gain/1
  Mux/1 -> Scope3/3
  Gain/1 -> Scope3/2, [P_BusDC]  "Power (kW)"

== system Model_14Bus_AC_DC_Microgrid/Bus_AC//DC4 ==
  note: C
  note: B
  note: A
  note: C
  note: Linea - Neutro
  note: B
  note: A
  note: C
  note: B
  note: A
  Conv pu1 : Gain  Gain=sqrt (3) /Vnom_ter_AC_DC  SaturateOnIntegerOverflow=on  OutDataTypeStr=Inherit: Same as input  ParamDataTypeStr=Inherit: Same as input
  Conv pu2 : Gain  Gain=sqrt (3) /Vnom_ter_AC_DC  SaturateOnIntegerOverflow=on  OutDataTypeStr=Inherit: Same as input  ParamDataTypeStr=Inherit: Same as input
  Measurement1 : Scope  NumInputPorts=4
      settings: SampleTime=Ts  Title=Active Powers (W)  ActiveDisplayYMinimum=-629.52557  ActiveDisplayYMaximum=1198.16221  DataLoggingVariableName=ScopeData8  DataLoggingSaveFormat=Array
  PLL : Subsystem
  PLL (3ph) : spsPLL3phLib/PLL (3ph)  Fmin=45  Par_Init=[0, 60]  ParK=[180, 3200, 1]  TcD=1e-4  MaxRateChangeFreq=12  FilterCutOffFreq=25  Ts=0  AGC=on
  Power Factor Block1 : Subsystem  mask(Power Factor Block){Freq=Fnom, Vinit=[0, 0], Iinit=[0, 0], Ts=0}
      mask prompts: Freq "Fundamental frequency (Hz):"; Vinit "Voltage initial input [ Mag, Phase (degrees) ]:"; Iinit "Current initial input [ Mag, Phase (degrees) ]:"; Ts "Sample time:"
      mask help:
      | Power Factor Block developed by Dr Rodney Tan
      | Version 1.01 (Aug 2016)
      |
      | Compute power factor and phase angle of AC circuit voltage-current pair at fundamental frequency.
      |
      | The computation is based on Power block and Complex number function block.
      |
      | For the first cycle of simulation, the outputs are held constant to the powers computed for the Voltage initial input and Current initial input parameters.
      mask Help:
      | <b>Fundamental Frequency (Hz)</b>
      | Specify the measurement fundamental frequency, in hertz, of the input signal.
      | 
      | <b>Voltage initial input [ Mag, Phase (degrees) ]</b>
      | Specify the voltage initial magnitude and phase to set a constant output for the first cycle of simulation.
      | 
      | <b>Current initial input [ Mag, Phase (degrees) ]</b>
      | Specify the current initial magnitude and phase to set a constant output for the first cycle of simulation.
      | 
      | <b>Sample Time</b>
      | Specify the sample time of the block, in seconds. Set to 0 to implement a continuous block.
      mask TypeOptions Freq: Power/Freq
      mask TypeOptions Vinit: Power/Vinit
      mask TypeOptions Iinit: Power/Iinit
      mask TypeOptions Ts: Power/Ts
  Power Factor1 : Display
  Scope : Scope
      settings: ActiveDisplayYMinimum=-60.85907  ActiveDisplayYMaximum=239.33693  DataLoggingVariableName=ScopeData5
  Scope1 : Scope
      settings: ActiveDisplayYMinimum=-0.59192  ActiveDisplayYMaximum=1.17688
  Scope2 : Scope
      settings: DataLoggingVariableName=ScopeData9
  THD : spsTHDLib/THD  Freq=60  Ts=Ts_Power
  THD (% and signal) : Scope  NumInputPorts=2
      settings: TimeSpan=0.1  ActiveDisplayYMinimum=-207.38986  ActiveDisplayYMaximum=214.23912  DataLoggingVariableName=ScopeData17
  THD (%) : Display
      settings: Format=bank
  Terminator : Terminator
  Vabc pu1 : Scope
      settings: TimeSpan=3  Title=Vabc_Instantaneo y rms (pu)  ActiveDisplayYMinimum=-2.15654  ActiveDisplayYMaximum=2.48621  DataLoggingVariableName=ScopeData10
  frecuency (Hz) : Display
  to % : Gain  Gain=100  SampleTime=Ts_Power
  ángulo de V (%)1 : Display
      settings: Format=bank
  wires:
  [Iabc_B1_busDC1] -> Power Factor Block1/2(Iabc)
  THD/1 -> to %/1
  to %/1 -> THD (%)/1, THD (% and signal)/2  "THD (%)"
  Power Factor Block1/4(Iabc y Iabc (rms)) -> Measurement1/4
  Power Factor Block1/1(Pabc) -> Measurement1/1
  Conv pu1/1 -> Vabc pu1/1
  Power Factor Block1/5("PFabc ") -> Scope1/1, Power Factor1/1
  Power Factor Block1/2(Qabc) -> Measurement1/2
  Power Factor Block1/3(Vabc y Vabc (rms)) -> Conv pu1/1, Measurement1/3
  PLL/1(delta_abc) -> Scope/1, ángulo de V (%)1/1
  Conv pu2/1 -> PLL/1(Vabc_LN_pu)
  PLL (3ph)/2 -> Terminator/1
  [Vabc_B1_busDC1] -> PLL (3ph)/1, Conv pu2/1, THD/1, THD (% and signal)/1, Power Factor Block1/1(Vabc)  "Vabc"
  PLL (3ph)/1 -> Scope2/1, frecuency (Hz)/1

== system Model_14Bus_AC_DC_Microgrid/Bus_AC//DC5 ==
  note: C
  note: B
  note: A
  note: C
  note: Linea - Neutro
  note: B
  note: A
  note: B
  note: C
  note: A
  Conv pu1 : Gain  Gain=sqrt (3) /Vnom_ter_AC_DC  SaturateOnIntegerOverflow=on  OutDataTypeStr=Inherit: Same as input  ParamDataTypeStr=Inherit: Same as input
  Conv pu2 : Gain  Gain=sqrt (3) /Vnom_ter_AC_DC  SaturateOnIntegerOverflow=on  OutDataTypeStr=Inherit: Same as input  ParamDataTypeStr=Inherit: Same as input
  Measurement1 : Scope  NumInputPorts=4
      settings: SampleTime=Ts  Title=Active Powers (W)  ActiveDisplayYMinimum=-361.73977  ActiveDisplayYMaximum=1065.47769  DataLoggingVariableName=ScopeData11  DataLoggingSaveFormat=Array
  PLL : Subsystem
  PLL (3ph) : spsPLL3phLib/PLL (3ph)  Fmin=45  Par_Init=[0, 60]  ParK=[180, 3200, 1]  TcD=1e-4  MaxRateChangeFreq=12  FilterCutOffFreq=25  Ts=0  AGC=on
  Power Factor Block1 : Subsystem  mask(Power Factor Block){Freq=Fnom, Vinit=[0, 0], Iinit=[0, 0], Ts=0}
      mask prompts: Freq "Fundamental frequency (Hz):"; Vinit "Voltage initial input [ Mag, Phase (degrees) ]:"; Iinit "Current initial input [ Mag, Phase (degrees) ]:"; Ts "Sample time:"
      mask help:
      | Power Factor Block developed by Dr Rodney Tan
      | Version 1.01 (Aug 2016)
      |
      | Compute power factor and phase angle of AC circuit voltage-current pair at fundamental frequency.
      |
      | The computation is based on Power block and Complex number function block.
      |
      | For the first cycle of simulation, the outputs are held constant to the powers computed for the Voltage initial input and Current initial input parameters.
      mask Help:
      | <b>Fundamental Frequency (Hz)</b>
      | Specify the measurement fundamental frequency, in hertz, of the input signal.
      | 
      | <b>Voltage initial input [ Mag, Phase (degrees) ]</b>
      | Specify the voltage initial magnitude and phase to set a constant output for the first cycle of simulation.
      | 
      | <b>Current initial input [ Mag, Phase (degrees) ]</b>
      | Specify the current initial magnitude and phase to set a constant output for the first cycle of simulation.
      | 
      | <b>Sample Time</b>
      | Specify the sample time of the block, in seconds. Set to 0 to implement a continuous block.
      mask TypeOptions Freq: Power/Freq
      mask TypeOptions Vinit: Power/Vinit
      mask TypeOptions Iinit: Power/Iinit
      mask TypeOptions Ts: Power/Ts
  Power Factor1 : Display
  Scope : Scope
      settings: ActiveDisplayYMinimum=-60.00715  ActiveDisplayYMaximum=239.87716  DataLoggingVariableName=ScopeData6
  Scope1 : Scope
      settings: ActiveDisplayYMinimum=-1.24821  ActiveDisplayYMaximum=1.2498  DataLoggingVariableName=ScopeData2
  Scope2 : Scope
      settings: DataLoggingVariableName=ScopeData10
  THD : spsTHDLib/THD  Freq=60  Ts=Ts_Power
  THD (% and signal) : Scope  NumInputPorts=2
      settings: TimeSpan=0.1  ActiveDisplayYMinimum=-21318.64578  ActiveDisplayYMaximum=21318.87173  DataLoggingVariableName=ScopeData18
  THD (%) : Display
      settings: Format=bank
  Terminator : Terminator
  Vabc pu1 : Scope
      settings: TimeSpan=3  Title=Vabc_Instantaneo y rms (pu)  ActiveDisplayYMinimum=-1.69301  ActiveDisplayYMaximum=1.69231  DataLoggingVariableName=ScopeData12
  frecuency (Hz) : Display
  to % : Gain  Gain=100  SampleTime=Ts_Power
  ángulo de V (%)1 : Display
      settings: Format=bank
  wires:
  [Iabc_B1_busDC2] -> Power Factor Block1/2(Iabc)
  THD/1 -> to %/1
  to %/1 -> THD (%)/1, THD (% and signal)/2  "THD (%)"
  Power Factor Block1/4(Iabc y Iabc (rms)) -> Measurement1/4
  Power Factor Block1/1(Pabc) -> Measurement1/1
  Conv pu1/1 -> Vabc pu1/1
  Power Factor Block1/5("PFabc ") -> Scope1/1, Power Factor1/1
  Power Factor Block1/2(Qabc) -> Measurement1/2
  Power Factor Block1/3(Vabc y Vabc (rms)) -> Conv pu1/1, Measurement1/3
  Conv pu2/1 -> PLL/1(Vabc_LN_pu)
  PLL/1(delta_abc) -> Scope/1, ángulo de V (%)1/1
  PLL (3ph)/2 -> Terminator/1
  [Vabc_B1_busDC2] -> Power Factor Block1/1(Vabc), PLL (3ph)/1, Conv pu2/1, THD/1, THD (% and signal)/1  "Vabc"
  PLL (3ph)/1 -> Scope2/1, frecuency (Hz)/1
